simulink model "insulinGlucoseSimHumanCtrl_00"  (Simulink 7.5)
settings: Solver=ode45  StartTime=0.0  StopTime=400  RelTol=1e-3
PreLoadFcn:
  | calibError = 0;
  | sTime_announce = 40;
  | mDuration_announce = 30;
  | carbs_announce = 200;
  | gi_announce = 40;
  | correctionBolusTime = 150;
  | sTime_actual = 40;
  | mDuration_actual = 30;
  | carbs_actual = 200;
  | gi_actual = 40;
libraries: dspsigops x1
settings Model: Creator=indriagobal  LastModifiedBy=indriagobal  SimulationMode=accelerator  TunableVars=calibError,carbs_actual,carbs_announce,correctionBolusTime,gi_actual,gi_announce,mDuration_actual,mDuration_announce,sTime_actual,sTime_announce  TunableVarsStorageClass=Auto,Auto,Auto,Auto,Auto,Auto,Auto,Auto,Auto,Auto  TunableVarsTypeQualifier=,,,,,,,,,
settings SolverCC: MaxConsecutiveZCs=100
settings DataIOCC: LimitDataPoints=off  SaveFormat=StructureWithTime  SaveOutput=off  SignalLogging=off  DSMLogging=off  SaveTime=off
settings OptimizationCC: InlineParams=on
settings DebuggingCC: SolverPrmCheckMsg=none

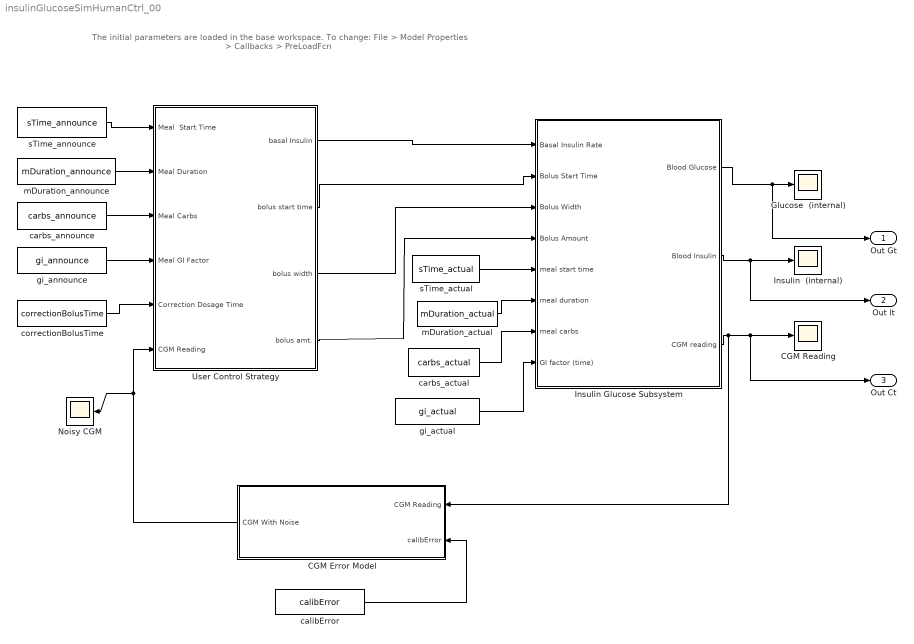
== system insulinGlucoseSimHumanCtrl_00 ==
  note: The initial parameters are loaded in the base workspace.
      | To change: File > Model Properties > Callbacks > PreLoadFcn
  CGM Error Model : Subsystem
  CGM Reading : Scope
      settings: YMin=0  YMax=12  SaveName=ScopeData3
  Glucose  (internal) : Scope
      settings: YMin=0  YMax=12  SaveName=ScopeData5
  Insulin  (internal) : Scope
      settings: YMin=0  YMax=0.1  SaveName=ScopeData6
  Insulin Glucose Subsystem : Subsystem
  Noisy CGM : Scope
      settings: YMin=0  YMax=12
  User Control Strategy : Subsystem
  calibError : Constant  Value=calibError
  carbs_actual : Constant  Value=carbs_actual
  carbs_announce : Constant  Value=carbs_announce
  correctionBolusTime : Constant  Value=correctionBolusTime
  gi_actual : Constant  Value=gi_actual
  gi_announce : Constant  Value=gi_announce
  mDuration_actual : Constant  Value=mDuration_actual
  mDuration_announce : Constant  Value=mDuration_announce
  sTime_actual : Constant  Value=sTime_actual
  sTime_announce : Constant  Value=sTime_announce
  Out Gt : Outport
  Out lt : Outport  Port=2
  Out Ct : Outport  Port=3
  wires:
  Insulin Glucose Subsystem/1(Blood Glucose) -> Glucose  (internal)/1, Out Gt/1
  Insulin Glucose Subsystem/3(CGM reading) -> CGM Error Model/1(CGM Reading), CGM Reading/1, Out Ct/1
  CGM Error Model/1(CGM With Noise) -> User Control Strategy/6(CGM Reading), Noisy CGM/1
  User Control Strategy/1(basal Insulin) -> Insulin Glucose Subsystem/1(Basal Insulin Rate)
  User Control Strategy/2(bolus start time) -> Insulin Glucose Subsystem/2(Bolus Start Time)
  User Control Strategy/3(bolus width) -> Insulin Glucose Subsystem/3(Bolus Width)
  User Control Strategy/4(bolus amt.) -> Insulin Glucose Subsystem/4(Bolus Amount)
  sTime_announce/1 -> User Control Strategy/1(Meal  Start Time)
  mDuration_announce/1 -> User Control Strategy/2(Meal Duration)
  carbs_announce/1 -> User Control Strategy/3(Meal Carbs)
  gi_announce/1 -> User Control Strategy/4(Meal GI Factor)
  Insulin Glucose Subsystem/2(Blood Insulin) -> Insulin  (internal)/1, Out lt/1
  sTime_actual/1 -> Insulin Glucose Subsystem/5(meal start time)
  mDuration_actual/1 -> Insulin Glucose Subsystem/6(meal duration)
  carbs_actual/1 -> Insulin Glucose Subsystem/7(meal carbs)
  gi_actual/1 -> Insulin Glucose Subsystem/8(GI factor (time))
  calibError/1 -> CGM Error Model/2(calibError)
  correctionBolusTime/1 -> User Control Strategy/5(Correction Dosage Time)

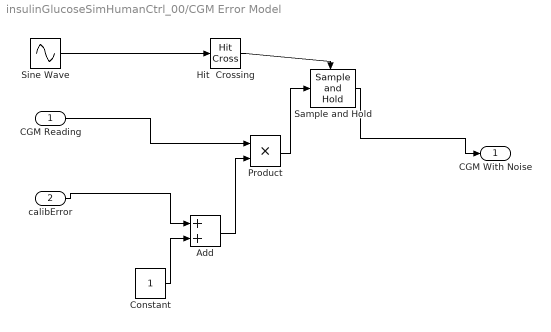
== system insulinGlucoseSimHumanCtrl_00/CGM Error Model ==
  CGM Reading : Inport
  calibError : Inport  Port=2
  Add : Sum
  Constant : Constant
  Hit  Crossing : HitCross  HitCrossingDirection=rising
  Product : Product  RndMeth=Zero
  Sample and Hold : dspsigops/Sample and Hold  SystemSampleTime=-1  trig=Rising edge  initCond=4.0  latchinput=off
  Sine Wave : Sin  Amplitude=1  Bias=0  Frequency=2 * 3.1415/20  Phase=0  Samples=10  SampleTime=0  Offset=0
  CGM With Noise : Outport
  wires:
  calibError/1 -> Add/1
  Constant/1 -> Add/2
  Add/1 -> Product/2
  Product/1 -> Sample and Hold/1
  CGM Reading/1 -> Product/1
  Sample and Hold/1 -> CGM With Noise/1
  Sine Wave/1 -> Hit  Crossing/1
  Hit  Crossing/1 -> Sample and Hold/Trigger

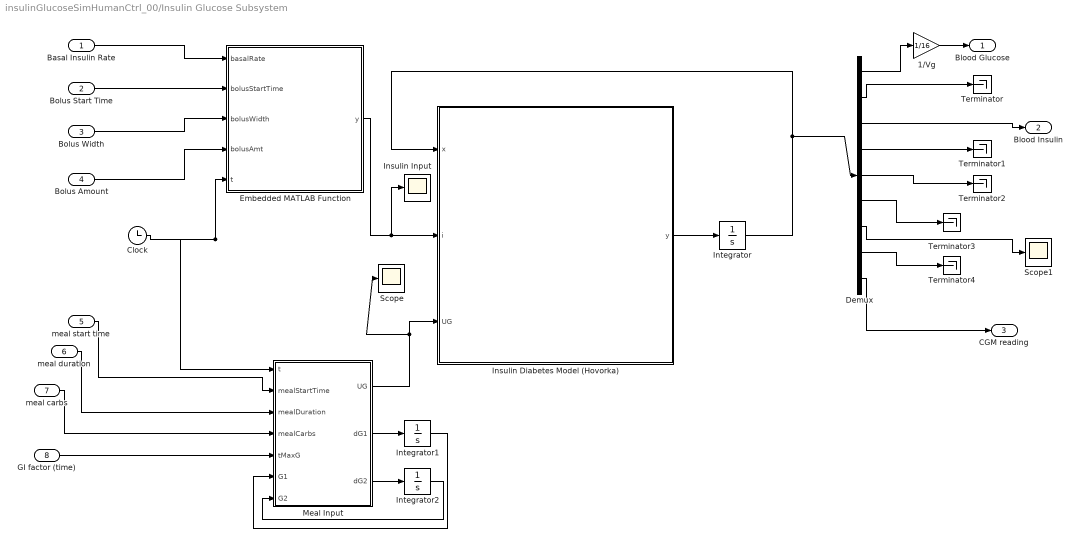
== system insulinGlucoseSimHumanCtrl_00/Insulin Glucose Subsystem ==
  Basal Insulin Rate : Inport
  Bolus Start Time : Inport  Port=2
  Bolus Width : Inport  Port=3
  Bolus Amount : Inport  Port=4
  meal start time : Inport  Port=5
  meal duration : Inport  Port=6
  meal carbs : Inport  Port=7
  GI factor (time) : Inport  Port=8
  1/Vg : Gain  Gain=1/16
  Clock : Clock
      settings: Decimation=1000
  Demux : Demux  Outputs=9
  Embedded MATLAB Function : Stateflow chart  TreatAsAtomicUnit=on
  Insulin Diabetes Model (Hovorka) : Stateflow chart  TreatAsAtomicUnit=on
  Insulin Input : Scope
      settings: YMin=0  YMax=2.5  SaveName=ScopeData4
  Integrator : Integrator  InitialCondition=[64.0; 40.0; 0.03 ; 0.03; 0.045; 0.04; 4.2; 4; 4]
  Integrator1 : Integrator
  Integrator2 : Integrator
  Meal Input : Stateflow chart  TreatAsAtomicUnit=on
  Scope : Scope
  Scope1 : Scope
      settings: SaveName=ScopeData7
  Terminator{,1..4} (5 alike) : Terminator
  Blood Glucose : Outport
  Blood Insulin : Outport  Port=2
  CGM reading : Outport  Port=3
  wires:
  Insulin Diabetes Model (Hovorka)/1(y) -> Integrator/1
  Integrator/1 -> Insulin Diabetes Model (Hovorka)/1(x), Demux/1
  Clock/1 -> Meal Input/1(t), Embedded MATLAB Function/5(t)
  Embedded MATLAB Function/1(y) -> Insulin Diabetes Model (Hovorka)/2(i), Insulin Input/1
  Demux/3 -> Blood Insulin/1
  Demux/1 -> 1/Vg/1
  1/Vg/1 -> Blood Glucose/1
  Demux/9 -> CGM reading/1
  meal start time/1 -> Meal Input/2(mealStartTime)
  meal duration/1 -> Meal Input/3(mealDuration)
  meal carbs/1 -> Meal Input/4(mealCarbs)
  Basal Insulin Rate/1 -> Embedded MATLAB Function/1(basalRate)
  Bolus Start Time/1 -> Embedded MATLAB Function/2(bolusStartTime)
  Bolus Width/1 -> Embedded MATLAB Function/3(bolusWidth)
  Bolus Amount/1 -> Embedded MATLAB Function/4(bolusAmt)
  Meal Input/1(UG) -> Insulin Diabetes Model (Hovorka)/3(UG), Scope/1
  Meal Input/2(dG1) -> Integrator1/1
  Meal Input/3(dG2) -> Integrator2/1
  Integrator2/1 -> Meal Input/7(G2)
  Integrator1/1 -> Meal Input/6(G1)
  GI factor (time)/1 -> Meal Input/5(tMaxG)
  Demux/7 -> Scope1/1
  Demux/2 -> Terminator/1
  Demux/4 -> Terminator1/1
  Demux/5 -> Terminator2/1
  Demux/6 -> Terminator3/1
  Demux/8 -> Terminator4/1

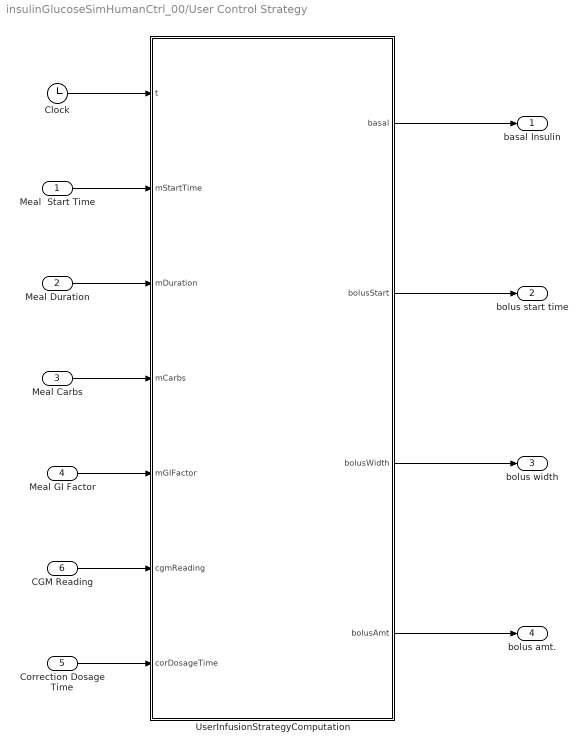
== system insulinGlucoseSimHumanCtrl_00/User Control Strategy ==
  Meal  Start Time : Inport
  Meal Duration : Inport  Port=2
  Meal Carbs : Inport  Port=3
  Meal GI Factor : Inport  Port=4
  Correction Dosage Time : Inport  Port=5
  CGM Reading : Inport  Port=6
  Clock : Clock
      settings: Decimation=10
  UserInfusionStrategyComputation : Stateflow chart  TreatAsAtomicUnit=on
  basal Insulin : Outport
  bolus start time : Outport  Port=2
  bolus width : Outport  Port=3
  bolus amt. : Outport  Port=4
  wires:
  Clock/1 -> UserInfusionStrategyComputation/1(t)
  Meal  Start Time/1 -> UserInfusionStrategyComputation/2(mStartTime)
  Meal Duration/1 -> UserInfusionStrategyComputation/3(mDuration)
  Meal Carbs/1 -> UserInfusionStrategyComputation/4(mCarbs)
  Meal GI Factor/1 -> UserInfusionStrategyComputation/5(mGIFactor)
  Correction Dosage Time/1 -> UserInfusionStrategyComputation/7(corDosageTime)
  CGM Reading/1 -> UserInfusionStrategyComputation/6(cgmReading)
  UserInfusionStrategyComputation/1(basal) -> basal Insulin/1
  UserInfusionStrategyComputation/2(bolusStart) -> bolus start time/1
  UserInfusionStrategyComputation/3(bolusWidth) -> bolus width/1
  UserInfusionStrategyComputation/4(bolusAmt) -> bolus amt./1

== matlab function Insulin Glucose Subsystem/Meal Input ==
  data: UG output double; t input double; dG1 output double; mealStartTime input double; mealDuration input double; mealCarbs input double; tMaxG input double; G1 input double; G2 input double; dG2 output double
function [UG,dG1,dG2] = mealInput(t,mealStartTime, mealDuration, mealCarbs,tMaxG, G1,G2)
% mealInput: Obtain the meal glucose input as a function of time given 
%   t : current simulation time
%   mealStartTime: when did the meal start
%   mealDuration: what is the meal duration.
%   mealCarbs: how many gms of carbs in the meal


y = 0.0; %% default output
fTimeVec = [0.0; 0.2; 0.8; 1.0];
fCarbVec = [0.5; 0.8/0.6; 0.5; 0.0 ];
tp = (t - mealStartTime)/mealDuration;
if (tp < 0.0 || tp > 1.0) 
    y = 0.0;
else 
    [m ~] = size(fTimeVec);
    for i = 1:(m-1)
    
       if ((tp >= fTimeVec(i,1)) && ( tp < fTimeVec(i+1,1)))
           y = fCarbVec(i,1) * mealCarbs/mealDuration; 
       end
    end
end

DG = y;
AG = 0.8; %% bio availability of carbohydrates

%% Gut absorption submodel
dG1 = - G1/tMaxG + AG * DG; %% dG1/dt
dG2 = G1/tMaxG - G2/tMaxG; %% dG2/dt
UG = G2/tMaxG;

== matlab function Insulin Glucose Subsystem/Insulin Diabetes Model (Hovorka) ==
  data: y output double; x input double; i input double; UG input double
function y = insulinGlucoseSimulinkBlkFun(x,i,UG)

%% De Model Constants
w = 100; %% Patient weight (kg)
k12 = 0.066; %% Transfer rate for insulin
ka1 = 0.006; %% deactivation rate for insulin transport
ka2 = 0.06; %% deactivation rate for insulin EGP
ka3 = 0.03; %% deactivation rate for insulin ??
kb1=0.0034;
kb2=0.056;
kb3=0.024;
ke = 0.138; %% insulin elimination from plasma
VI = 0.12 * w; %% insulin distrib volume
VG = 0.16 * w; %% glucose distrib volume

Sf1T = 51.2 * 0.0001;
Sf1D = 8.2 * 0.0001;
Sf1E = 520 * 0.0001;
EGP0 = 0.0161*w;
F01 = 0.0097*w;
tMaxI=55;
kaInt = 0.05;

%%

q1 = x(1,1);
q2 = x(2,1);
I = x(3,1);
x1 = x(4,1);
x2 = x(5,1);
x3 = x(6,1);
s1 = x(7,1);
s2 = x(8,1);
C = x(9,1);
%%G1 = x(10,1);
%%G2 = x(11,1);


y = zeros(9,1);

EGP = max (0.0, EGP0 * (1 + x3));




G = q1/VG;

%% From Chee and Fernando book
% if ( G >= 4.5) 
%     F01c = F01;
% else
%     F01c = F01 * G /4.5;
% end

%% From Wilinska et al. J. Diabetes Sci and Tech. Jan 2010

F01c = F01 * G/(G + 1) / 0.85;

if ( G >= 9)
    Fr = 0.003 * (G - 9) * VG;
else
    Fr = 0;
end

u = i;

%% Divide input glucode UG by 180 to convert to mol. Since UG is in grams, multiply by 1000 to get milli moles
y(1,1) =  - ( F01c + x1 * q1) + k12 * q2 - Fr + EGP + UG/180*1000 ; %% dq1/dt;
y(2,1) = x1 * q1 - (k12 + x2) * q2; %% dq2/dt

y(4,1) = - ka1 * x1 + kb1 * I; %% dx1/dt
y(5,1) = - ka2 * x2 + kb2 * I; %% dx2/dt
y(6,1) = - ka3 * x3 + kb3 * I; %% dx3/dt

%% Insulin Action submodel.
y(3,1) = s2/(tMaxI * VI) - ke * I; %% dI/dt  %% Note ka = 1 / tMaxI
y(7,1) = u - s1/tMaxI; %%ds1/dt
y(8,1) = s1/tMaxI - s2/tMaxI; %% ds2/dt

%% Subcutaneous glucose transfer: modeling first order lag
y(9,1) = kaInt * ( G - C); %% dc/dt 

%% Gut absorption submodel
%%y(10,1) = - G1/tMaxG + AG * DG; %% dG1/dt
%% y(11,1) = G1/tMaxG - G2/tMaxG; %% dG2/dt





end

== matlab function Insulin Glucose Subsystem/Embedded MATLAB Function ==
  data: basalRate input double; bolusStartTime input double; bolusWidth input double; bolusAmt input double; t input double; y output double
function y = insulinPump(basalRate, bolusStartTime, bolusWidth, bolusAmt,t)
%% insulinInfusionPump: Simulate the action of an insulin infusion pump roughly 
%%    basalRate: the basal infusion rate
%%    bolusStartTime:  if this is  > 0 then it specifies when the bolus should be started.
%%    bolusWidth: how long should the bolus last
%%    bolusAmt: what should the bolus amount be

y = basalRate;

if (bolusStartTime < -1)
 return ;
end

tp = (t - bolusStartTime)/bolusWidth;

if ((tp < 0) || (tp >1))
    return;
end

tProf = [0; 0.1; 0.2; 0.3; 0.4;0.5; 0.6; 0.7; 0.8; 0.9; 1.0];
[m ~] = size(tProf);
iProf = [0.25; %% 0.025 
         0.5; %% 0.075
         1.0; %% 0.175
         1.5; %% 0.325
         3.0; %% 0.625
         1.5; %% 0.775
         1.0; %% 0.875
         0.5; %% 0.925
         0.25; %% 0.95
         0.2 ; %% 0.97
         ];
     
for i = 1:(m-1)
    if (tp >= tProf(i,1) && tp < tProf(i+1,1))
        y = y + iProf(i,1) * bolusAmt/bolusWidth;
        return ;
    end
end

== matlab function User Control Strategy/UserInfusionStrategyComputation ==
  data: t input double; basal output double; mStartTime input double; mDuration input double; mCarbs input double; mGIFactor input double; cgmReading input double; corDosageTime input double; bolusStart output double; bolusWidth output double; bolusAmt output double
function [basal,bolusStart, bolusWidth,bolusAmt] =  computeUserInfusionStrategy(t, mStartTime, mDuration, mCarbs, mGIFactor, cgmReading, corDosageTime)
%% function computeUserInfusionStrategy
%% compute the basal insulin, bolus start time, bolus width, bolus amount, meal start time 
%% t = current simulation time
%% mStartTime: meal starting time.
%% mDuration: meal duration
%% mGIFactor: meal GI factor
%% cgmReading:  CGM reading
%% corDosageTime: correction dosage time


%% Assume users intende and actual meal data are identical for now.
%% Todo: investigate the possibility of adding errors here later.

icRatio = 0.1386; %% patient's insulin to carbs ratio

basal = 0.08;

bolusStart = 0;
bolusWidth=0;
bolusAmt =0;
if ( t < corDosageTime)   
    bolusAmt = mCarbs * icRatio;
    bolusStart = max(0, mStartTime -40 );
    bolusWidth = 16.6;  
else 
   
       if (cgmReading > 8.0)
          bolusStart = corDosageTime + 10.0;
          bolusAmt = (cgmReading - 8.0)*10.0/74.0;
          bolusWidth = 10;
          return;
       end
end
